simulink model "usrp_4t12r_heatmap"  (R2018a)
settings: Solver=VariableStepDiscrete  StartTime=0.0  StopTime=inf  RelTol=1e-3
undefined symbols (not defined in the file): fft2, gather, get, gpuArray, parula, psBcoor, psWcen, rfcaptureC2Fsim, Time, tsRamp, us
libraries: neural x14, visionanalysis x8, dspobslib x8, dspfdesign x7, dspstat3 x5, dspbuff3 x2, visionsinks x2, commsdrhw_v2 x1, visiontextngfix x1, dspvision x1, visiontransforms x1, dspsigops x1
(part 4 of 4)

== system usrp_4t12r_heatmap/定位系统/定位模块/Pattern Recognition Neural Network1/Layer 2/Delays 1 ==
  "p{2}" : Inport  PortDimensions=10
      mask Display: e = 0.06;c1 = [120 230 180]/255;c2 = ([120 230 180]+0)/(256+128);c3 = ([120 230 180]+128)/(256+128);patch([0 1 1 0],[0 0 1 1],c1);patch([0 1 1 1-e 1-e 0+e],[0 0 1 1-e 0+e 0+e],c2);patch([0 0 1 1-e 0+e 0+e],[0 1 1 1-e 1-e 0+e],c3);plot([0 1 1 0 0],[0 0 1 1 0]);
  mux : Mux  Inputs=1
      mask Display: e = 0.06;c1 = [120 150 230]/255;c2 = ([120 150 230]+0)/383;c3 = ([120 150 230]+128)/383;patch([0 1 1 0],[0 0 1 1],c1);patch([0 1 1 1-e 1-e 0+e],[0 0 1 1-e 0+e 0+e],c2);patch([0 0 1 1-e 0+e 0+e],[0 1 1 1-e 1-e 0+e],c3);plot([0 1 1 0 0],[0 0 1 1 0]);disp('Mux')
  "pd{2,1}" : Outport
      mask Display: e = 0.06;c1 = [120 230 180]/255;c2 = ([120 230 180]+0)/(256+128);c3 = ([120 230 180]+128)/(256+128);patch([0 1 1 0],[0 0 1 1],c1);patch([0 1 1 1-e 1-e 0+e],[0 0 1 1-e 0+e 0+e],c2);patch([0 0 1 1-e 0+e 0+e],[0 1 1 1-e 1-e 0+e],c3);plot([0 1 1 0 0],[0 0 1 1 0]);
  wires:
  "p{2}"/1 -> mux/1
  mux/1 -> "pd{2,1}"/1

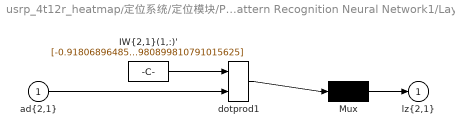
== system usrp_4t12r_heatmap/定位系统/定位模块/Pattern Recognition Neural Network1/Layer 2/LW{2,1} ==
  "ad{2,1}" : Inport  PortDimensions=10
      mask Display: e = 0.06;c1 = [120 230 180]/255;c2 = ([120 230 180]+0)/(256+128);c3 = ([120 230 180]+128)/(256+128);patch([0 1 1 0],[0 0 1 1],c1);patch([0 1 1 1-e 1-e 0+e],[0 0 1 1-e 0+e 0+e],c2);patch([0 0 1 1-e 0+e 0+e],[0 1 1 1-e 1-e 0+e],c3);plot([0 1 1 0 0],[0 0 1 1 0]);
  "IW{2,1}(1,:)'" : Constant  Value=[-0.9180689648575157679744052074966020882129669189453125;-1.2325699044823650307733942099730484187602996826171875;-0.433230835269282132937718188259168528020381927490234375;1.070049805355919314564516753307543694972991943359375;1.348178691344017021691570334951393306255340576171875;1.3397600801852520557844172799377702176570892333984375;-1.0018158100448253389203046026523225009441375732421875;-0.2030426599098004991628130255776341073215007781982421875;0.9292484845906765489331746721290983259677886962890625;-1.1503127318623340702430368764908052980899810791015625]
      mask Display: e = 0.06;c1 = [120 150 230]/255;c2 = ([120 150 230]+0)/383;c3 = ([120 150 230]+128)/383;patch([0 1 1 0],[0 0 1 1],c1);patch([0 1 1 1-e 1-e 0+e],[0 0 1 1-e 0+e 0+e],c2);patch([0 0 1 1-e 0+e 0+e],[0 1 1 1-e 1-e 0+e],c3);plot([0 1 1 0 0],[0 0 1 1 0]);disp('weights');
  Mux : Mux  Inputs=1
      mask Display: e = 0.06;c1 = [120 150 230]/255;c2 = ([120 150 230]+0)/383;c3 = ([120 150 230]+128)/383;patch([0 1 1 0],[0 0 1 1],c1);patch([0 1 1 1-e 1-e 0+e],[0 0 1 1-e 0+e 0+e],c2);patch([0 0 1 1-e 0+e 0+e],[0 1 1 1-e 1-e 0+e],c3);plot([0 1 1 0 0],[0 0 1 1 0]);disp('Mux');
  dotprod1 : neural/Weight Functions/dotprod
  "lz{2,1}" : Outport
      mask Display: e = 0.06;c1 = [120 230 180]/255;c2 = ([120 230 180]+0)/(256+128);c3 = ([120 230 180]+128)/(256+128);patch([0 1 1 0],[0 0 1 1],c1);patch([0 1 1 1-e 1-e 0+e],[0 0 1 1-e 0+e 0+e],c2);patch([0 0 1 1-e 0+e 0+e],[0 1 1 1-e 1-e 0+e],c3);plot([0 1 1 0 0],[0 0 1 1 0]);
  wires:
  "IW{2,1}(1,:)'"/1 -> dotprod1/1
  "ad{2,1}"/1 -> dotprod1/2
  dotprod1/1 -> Mux/1
  Mux/1 -> "lz{2,1}"/1

== matlab function usrp_4t12r_heatmap/定位系统/定位模块/帧同步与切割/getAntNum ==
  data: ysTr input; tTr input; trThres input; iRx output; fSraw parameter; lPul parameter; nPul parameter; rxBits parameter; txBits parameter; iTx output; nTx parameter; nRx parameter
%% 判断触发时间对应同步信号的天线编号
% iRx: 接收天线编号
% iTx: 发射天线编号
% ysTr: 一帧triger信号
% tRamp: 斜坡开始时间，以第一个采样点为参考时间0
% fSraw: 原始采样率
% lPul: 一个脉冲/比特采样点数
% nPul: 脉冲/比特总数
% rxBits: 接收天线比特
% txBits: 发射天线比特
% trThres: 触发电平
% nRx: 接收天线数量
% nTx: 发射天线数量
function [iRx,iTx]=getAntNum(ysTr, tTr, trThres, fSraw, lPul, nPul, rxBits, txBits, nTx, nRx)
if isnan(tTr)
    iRx=nan;
    iTx=nan;
    return
end
%% 准备参数
nPulRx=size(rxBits,2);
nPulTx=size(txBits,2);

%% 抽取天线编号的比特电平
iBit1=ceil(tTr*fSraw+1.5*lPul)+1;

tsBits=linspace(iBit1,iBit1+lPul*(nPulRx+nPulTx-1),nPul-1);
isBits=mod(tsBits-1,length(ysTr))+1;
ysBits=ysTr(isBits)>trThres;
isRx=find(all(~xor(rxBits,repmat(ysBits(1:nPulRx)',nRx,1)),2),1);
isTx=find(all(~xor(txBits,repmat(ysBits(nPulRx+1:nPul-1)',nTx,1)),2),1);
if isempty(isRx)
    iRx=nan;
else
    iRx=isRx(1);%为simulink推理iRx大小提供帮助
end
if isempty(isTx)
    iTx=nan;
else
    iTx=isTx(1);%为simulink推理iTx大小提供帮助
end


end

== matlab function usrp_4t12r_heatmap/定位系统/定位模块/帧同步与切割/firstTrTime ==
  data: ysTr input; tFtr output; fSraw parameter; lRampRaw parameter; lPul parameter; nPul parameter; trEdge parameter; trThres input; nRx parameter; nTx parameter; nCyclePF parameter
%% 同步斜坡信号起始时间函数，返回所有斜坡信号起始时间点
% tFramp: 第一个斜坡开始时间，精确到采样时间之下，以第一个采样点为参考时间0
% ysTr: 一帧triger信号
% fSraw: 原始采样率
% lRampRaw: 一个斜坡的原始采样点数
% lPul: 一个脉冲/比特采样点数
% nPul: 脉冲/比特总数
% trEdge: 触发沿：1上升沿 0下降沿
% trThres: 触发电平
% nRx: 接收天线数量
% nTx: 发射天线数量
% nCyclePF: 每帧包含的天线扫描周期数
function tFtr=firstTrTime(ysTr, fSraw, lRampRaw, lPul, nPul, trEdge, trThres, nRx, nTx, nCyclePF)

if(mod(length(ysTr),lRampRaw)~=0)
    error('The length of frame is not integer multiple of the length of ramp .');
end

%% 分析第一个完整斜坡同步信号
%第一个完整斜坡同步信号触发沿位于1:lRamp,为了容错，扩大范围到1:lRamp+lPul*nPul
if(nRx*nTx*nCyclePF>1)
    isFramp=1:lRampRaw+lPul*nPul;%indexs first ramp
else
    isFramp=1:lRampRaw;
end
ysTrFf=ysTr(isFramp);%ys triger first ramp
isTr=[];
if trEdge==0
    isTr=find(ysTrFf(2:end)<trThres & ysTrFf(1:end-1)>=trThres)+1;%index triger first
else
    isTr=find(ysTrFf(2:end)>trThres & ysTrFf(1:end-1)<=trThres)+1;
end
iTrF=0;
if isempty(isTr)
    tFtr=nan;
    return
else
    iTrF=isTr(find([true,diff(isTr,1,1)'>lPul*nPul],1,'last'));%要求脉冲和比特总时长小于斜坡周期的一半,选取最后一个触发信号
end


%% 线性插值分析触发沿的精确时间
tFtr=interp1(double([ysTr(iTrF-1),ysTr(iTrF)]),double([iTrF-1,iTrF]-1)/fSraw,double(trThres));
end

== matlab function usrp_4t12r_heatmap/定位系统/定位模块/帧同步与切割/interpShiftScale1 ==
  data: vIn input; vOut output; dis input; scFac input; isDown parameter
%% 循环移位，通过线性插值实现小数位数的移位
% vOut: 输出向量
% vIn: 输入向量
% dis: 向右移位距离
function vOut=interpShiftScaleDownsample(vIn, dis, scFac, isDown)
    if isnan(dis)||isnan(scFac)
        vOut=vIn(isDown);
        return
    end
    isZeroBased=(0:length(vIn)-1)';
    dis=dis/scFac;
    if dis>=0
        iShift=floor(dis);
        iAdd=dis-iShift;
    else
        iShift=ceil(dis);
        iAdd=iShift-dis;
    end
    
    isShifted=circshift(isZeroBased,iShift);

    vOut=interp1(isZeroBased/scFac,vIn, ...
        isShifted(isDown)+iAdd,'linear','extrap');
end

== matlab function usrp_4t12r_heatmap/定位系统/定位模块/帧同步与切割/calcShiftDis ==
  data: iRx input; iTx input; dis output; tFtr input; lRampRaw parameter; fSraw parameter; nRx parameter; nTx parameter
%% 通过天线序号、时间偏移计算循环移位位移量
% dis: 位移量
% iAnt: 天线序号，从1开始
% tFtr: 第一个触发信号时间
% lRampRaw: 一个斜坡的原始采样点数
% fSraw: 原始采样率
% nRx: 接收天线数量
% nTx: 发射天线数量
function dis=calcShiftDis(iRx, iTx, tFtr, lRampRaw, fSraw, nRx, nTx)
    dis=-((nRx*nTx+1+nRx-iRx-nRx*iTx)*lRampRaw+(tFtr*fSraw));
end

== matlab function usrp_4t12r_heatmap/定位系统/定位模块/inPo2coor ==
  data: is input; coor output; dsVal parameter; angs parameter
function coor = isPo2coor(is, dsVal, angs)
coor=zeros(1,2,'single');
d=dsVal(is(1));
ang=angs(is(2));
coor(1)=d*sind(ang);
coor(2)=d*cosd(ang);

== matlab function usrp_4t12r_heatmap/定位系统/定位模块/帧同步与切割/calcTrThres ==
  data: ysTr input; trThres output
%% 计算触发电平
function trThres = calcTrThres(ysTr)
trThres=(max(ysTr)+min(ysTr))/2;%triger threshold
% trThres=(mean(ysTr(ysTr>trThres))+mean(ysTr(ysTr<trThres)))/2;
end

== matlab function usrp_4t12r_heatmap/定位系统/定位模块/热度图计算/MATLAB Function1 ==
  data: u input; y output
function y = fft2d(u)
y=fft2(u);

== matlab function usrp_4t12r_heatmap/定位系统/定位模块/热度图计算/heatMapShiftFlip ==
  data: u input; y output
function y = heatMapShiftFlip(u)
y =circshift(u,ceil(size(u,2)/2),2);
y=flip(y,2);

== matlab function usrp_4t12r_heatmap/定位系统/定位模块/帧同步与切割/scaleFactor ==
  data: ysTr input; tFTr input; trThres input; scFac output; fSraw parameter; fRamp parameter; trEdge parameter; nRx parameter; nTx parameter; nCyclePF parameter; ysTrLramp output
%% 同步斜坡信号起始时间函数，返回所有斜坡信号起始时间点
% scFac: 缩放因子，adf4159的时钟比usrp的时钟
% ysTrLramp: 输出最后一个触发沿的时域信号
% ysTr: 一帧triger信号
% tRamp: 斜坡开始时间，以第一个采样点为参考时间0
% trThres: 触发电平
% fSraw: 原始采样率
% fRamp: 斜坡频率
% trEdge: 触发沿：1上升沿 0下降沿
% nRx: 接收天线数量
% nTx: 发射天线数量
% nCyclePF: 每帧包含的天线扫描周期数
function [scFac, ysTrLramp]=scaleFactor(ysTr, tFTr, trThres, fSraw, fRamp, trEdge ,nRx, nTx, nCyclePF)
%% 准备参数
hW=ceil(nRx*nTx*nCyclePF*0.1);%half width

% 如果一个帧包含的ramp数小于3
% 可能导致无法定位最后一个ramp起始时间
% 因为tFramp可能识别为第一或二个ramp的起始时间
if isnan(tFTr) || nRx*nTx*nCyclePF<3
    scFac=nan;
    ysTrLramp=zeros(hW*2+1,1,'single');
    return
end

%% 根据第一个斜坡开始时间（tFramp）计算最后一个斜坡开始时间区间
iCen=round(tFTr*fSraw+fSraw/fRamp*(nRx*nTx*nCyclePF-2));
isLramp=(-hW:hW)+iCen;
ysTrLramp=ysTr(isLramp);

%% 分析最后一个斜坡开始时间
if trEdge==0
    isTr=find(ysTrLramp(2:end)<trThres & ysTrLramp(1:end-1)>=trThres)+1;%index triger first
else
    isTr=find(ysTrLramp(2:end)>trThres & ysTrLramp(1:end-1)<=trThres)+1;
end
iTrF=0;
if isempty(isTr)
    scFac=nan;
    ysTrLramp=zeros(hW*2+1,1,'single');
    return
else
    iTrF=isTr(1);
end

%% 线性插值分析触发沿的精确时间
tLramp=interp1(double([ysTrLramp(iTrF-1),ysTrLramp(iTrF)]),double([isLramp(iTrF)-1,isLramp(iTrF)]-1)/fSraw,double(trThres));
scFac=(tLramp-tFTr)*fRamp/(nRx*nTx*nCyclePF-2);
end

== matlab function usrp_4t12r_heatmap/定位系统/定位模块/rfcaptureC2F ==
  data: psWcen input size=[1,3]; psF output size=[length(ysF),length(xsF),length(zsF)]; psWl parameter; psWdC parameter; psBcoor parameter; psB parameter; C2Fratio parameter; C2Fw parameter; C2Fn parameter; rxCoor parameter; txCoor parameter; nRx parameter; nTx parameter; dCa parameter; tsRamp parameter; fBw parameter; fRamp parameter; dLambda parameter; yLoReshape input
%% rfcapture coarse to fine 函数。由粗到细计算功率分布

% psF: 精算功率分布, 实数

% psWcen: 窗口属性，结构体数组，包含xyz坐标、meshgrid、坐标
% psWcoor: 窗口中心坐标
% psBcoor: 背景坐标
% psB; 复数背景
% C2Fratio: coarse to fine 比例，选取C2Fratio*maxPower的点进行迭代
% tShowPsProject: 显示各精度投影图的间隔时间，为0时不显示
% hPs: 显示投影图的目标窗口句柄
% yLoReshape: 中频信号大小[length(tsRamp),nRx,nTx]
% rxCoor: 接收天线坐标
% txCoor: 发射天线座标
% nRx: 接收天线数量
% nTx: 发射天线数量
% dCa: 应减去的多余天线线缆距离
% tsRamp: 一个斜坡内的时间坐标
% fBw: 扫频带宽
% fRamp: 斜坡频率
% dLambda: 波长
% useGPU: 是否使用GPU

function psF=rfcaptureC2F(psWcen,psWl, psWdC, ...
    psBcoor,psB,C2Fratio,C2Fw, C2Fn, ...
    rxCoor, txCoor, nRx, nTx, dCa, tsRamp, fBw, fRamp, dLambda, yLoReshape)

% % 预分配内存
% preciFac=C2Fw^(C2Fn-1);
% psF=zeros(psWl(1)*preciFac/psWdC(1)+1, ...
%     psWl(2)*preciFac/psWdC(2)+1, ...
%     psWl(3)*preciFac/psWdC(3)+1, ...
%     'single');

% 最粗一级
xsC=single(-psWl(1)/2+psWcen(1):psWdC(1):psWl(1)/2+psWcen(1));
ysC=single(-psWl(2)/2+psWcen(2):psWdC(2):psWl(2)/2+psWcen(2));
zsC=single(-psWl(3)/2+psWcen(3):psWdC(3):psWl(3)/2+psWcen(3));

[xssC,yssC,zssC]=meshgrid(xsC,ysC,zsC);
psHcoor=[xssC(:),yssC(:),zssC(:)];
isHLog=true(size(xssC));
psF=zeros(size(xssC),'single');

for i=1:C2Fn

    % 抽取背景点
    isPsB=zeros(size(psHcoor,1),1);
    for j=1:size(psHcoor,1)
        isPsB(j)=find(all(abs( ...
            psBcoor-repmat(psHcoor(j,:),size(psBcoor,1),1) ...
            )<0.001,2),1);
    end
    psBH=psB(isPsB);

    % 硬算选取点
    fTsrampRTZ=rfcaptureCo2F(psHcoor,rxCoor,txCoor,nRx,nTx,dCa,tsRamp,fBw,fRamp,dLambda);
    psH=abs(rfcaptureF2ps(fTsrampRTZ,yLoReshape)-psBH);

    psF(isHLog)=psH;

    
    if i>=C2Fn
        break;
    end
    
    % 计算下一次迭代坐标
    xsF=single(-psWl(1)/2+psWcen(1):psWdC(1)/(C2Fw^i):psWl(1)/2+psWcen(1));
    ysF=single(-psWl(2)/2+psWcen(2):psWdC(2)/(C2Fw^i):psWl(2)/2+psWcen(2));
    zsF=single(-psWl(3)/2+psWcen(3):psWdC(3)/(C2Fw^i):psWl(3)/2+psWcen(3));
    
    [xssF,yssF,zssF]=meshgrid(xsF,ysF,zsF);
    coorF=[xssF(:),yssF(:),zssF(:)];
    
    % 扩展psF和isHLog矩阵
    psF=interp3(xssC,yssC,zssC, ...
        psF,xssF,yssF,zssF,'linear',0);
    
    % 根据规则选取精算点
    isHLog=psF>max(psF(:))*(1-C2Fratio);
    psHcoor=coorF(isHLog(:),:);
    
    xssC=xssF;
    yssC=yssF;
    zssC=zssF;
end

end

%% 根据rfcapture论文的硬算公式计算指定坐标上的功率大小

% fTsrampRTZ: 硬算公式的中间值f(n,m,zs,ts,tsRamp)，（ts为长时间,tsRamp为短时间）

% pointCoor: 指定坐标，n行3列
% rxCoor: 接收天线坐标
% txCoor: 发射天线座标
% nRx: 接收天线数量
% nTx: 发射天线数量
% dCa: 应减去的多余天线线缆距离
% tsRamp: 一个斜坡内的时间坐标
% fBw: 扫频带宽
% fRamp: 斜坡频率
% dLambda: 波长
% useGPU: 是否使用GPU

function fTsrampRTZ=rfcaptureCo2F(pointCoor,rxCoor,txCoor,nRx,nTx,dCa,tsRamp,fBw,fRamp,dLambda)
%% 计算r(n,m)(X(ts),Y(ts),z)，（ts为长时间）

nPair=nRx*nTx;
nP=size(pointCoor,1);
[isRx,isTx]=meshgrid(1:nRx,1:nTx);
isRx=permute(isRx,[2,1]);
isTx=permute(isTx,[2,1]);
isRxV=reshape(isRx,1,nPair);
isTxV=reshape(isTx,1,nPair);
rsCoRT=sqrt( ...
    (repmat(pointCoor(:,1),1,nPair)-repmat(rxCoor(isRxV,1)',nP,1)).^2 ...
    + (repmat(pointCoor(:,2),1,nPair)-repmat(rxCoor(isRxV,2)',nP,1)).^2 ...
    + (repmat(pointCoor(:,3),1,nPair)-repmat(rxCoor(isRxV,3)',nP,1)).^2 ...
    ) ...
    + sqrt( ...
    (repmat(pointCoor(:,1),1,nPair)-repmat(txCoor(isTxV,1)',nP,1)).^2 ...
    + (repmat(pointCoor(:,2),1,nPair)-repmat(txCoor(isTxV,2)',nP,1)).^2 ...
    + (repmat(pointCoor(:,3),1,nPair)-repmat(txCoor(isTxV,3)',nP,1)).^2 ...
    ) ...
    + dCa;
rsCoRT=reshape(rsCoRT,nP,nRx,nTx);

%% 计算f(n,m,zs,ts,tsRamp)，（ts为长时间,tsRamp为短时间）

rsCoRTTsramp=permute(repmat(rsCoRT,1,1,1,length(tsRamp)),[4,2,3,1]);
% persistent  tsCoRTTsramp;
tsCoRTTsramp=repmat(tsRamp',1,size(rsCoRTTsramp,2),size(rsCoRTTsramp,3),size(rsCoRTTsramp,4));
fTsrampRTZ=exp( ...
    1i*2*pi*fBw*fRamp.*rsCoRTTsramp/3e8 ...
    .*tsCoRTTsramp ...
    ) ...
    .*exp( ...
    1i*2*pi*rsCoRTTsramp/dLambda ...
    );
    
end

%% 根据rfcapture论文的硬算公式计算指定坐标上的功率大小

% ps: 对应点功率，复数

% fTsrampRTZ: 硬算公式的中间值f(n,m,zs,ts,tsRamp)，（ts为长时间,tsRamp为短时间）
% yLoReshape: 中频信号, 大小[length(tsRamp),nRx,nTx]
% useGPU: 是否使用GPU

function ps=rfcaptureF2ps(fTsrampRTZ,yLoReshape)
ps=shiftdim(sum(sum(sum(fTsrampRTZ.*repmat(yLoReshape,1,1,1,size(fTsrampRTZ,4)),1),2),3));
end

== matlab function usrp_4t12r_heatmap/定位系统/定位模块/帧同步与切割/interpShiftScale ==
  data: vIn input; vOut output; dis input; scFac input; isDown parameter
%% 循环移位，通过线性插值实现小数位数的移位
% vOut: 输出向量
% vIn: 输入向量
% dis: 向右移位距离
function vOut=interpShiftScaleDownsample(vIn, dis, scFac, isDown)
    if isnan(dis)||isnan(scFac)
        vOut=vIn(isDown);
        return
    end
    isZeroBased=(0:length(vIn)-1)';
    dis=dis/scFac;
    if dis>=0
        iShift=floor(dis);
        iAdd=dis-iShift;
    else
        iShift=ceil(dis);
        iAdd=iShift-dis;
    end
    
    isShifted=circshift(isZeroBased,iShift);

    vOut=interp1(isZeroBased/scFac,vIn, ...
        isShifted(isDown)+iAdd,'linear','extrap');
end

== matlab function usrp_4t12r_heatmap/定位系统/定位模块/MATLAB Function ==
  data: xy input; psWcen output; xsB parameter; ysB parameter; psWl parameter; zMa parameter; zMi parameter
function psWcen = getPsWcen(xy, xsB, ysB, psWl, zMa, zMi)
psWcen=zeros(1,3,'single');
xsB=xsB(xsB>=xsB(1)+psWl(1)/2 & xsB<=xsB(end)-psWl(1)/2);
ysB=ysB(ysB>=ysB(1)+psWl(2)/2 & ysB<=ysB(end)-psWl(2)/2);
psWcen(1)=interp1(xsB,xsB,xy(1),'nearest','extrap');
psWcen(2)=interp1(ysB,ysB,xy(2),'nearest','extrap');
psWcen(3)=(zMa+zMi)/2;
end

== matlab function usrp_4t12r_heatmap/定位系统/定位模块/calcShape ==
  data: xywl output; psWl parameter; dxF parameter; dyF parameter; psWcen input; xsB parameter; ysB parameter
function xywl = calcShape(psWl, dxF, dyF, psWcen, xsB, ysB)
iXTar=interp1(xsB,1:length(xsB),psWcen(1),'nearest');
iYTar=interp1(ysB,1:length(ysB),psWcen(2),'nearest');
lXW=psWl(1)/dxF;
lYW=psWl(2)/dyF;
xywl=[iXTar-lXW/2 iYTar-lYW/2 lXW lYW];

== matlab function usrp_4t12r_heatmap/定位系统/定位模块/heatMapPo2Car ==
  data: heatMapPo input; heatMapCar output; angs parameter; dsVal parameter; xsB parameter; ysB parameter
function heatMapCar = heatMapPo2Car(heatMapPo,angs, dsVal, xsB, ysB)
[xssB2,yssB2]=meshgrid(xsB,ysB);
heatMapCar=zeros(length(ysB),length(xsB),'single');
dsPo2Car=sqrt(xssB2.^2+yssB2.^2);
angsPo2Car=atand(xssB2./yssB2);
angsPo2Car(isnan(angsPo2Car))=0;
heatMapCar=interp2(angs,dsVal,heatMapPo,angsPo2Car,dsPo2Car,'linear',0);
